simulink model "simThreeLinkFTC"  (R2014b)
settings: Solver=ode45  StartTime=0.0  StopTime=tof  FixedStep=dt  MaxStep=dtmax  RelTol=1e-3
values from neighbouring files (symbols this model uses):
  alpha = 1    [robotArmWith2Links.m]    (also in threeLinkFTC.m; twoLinkFTC.m; twoLinkFTCwAdaptive.m)
  Ar = [0 5; -30 -30]    [robotArmWith2Links.m]    (also in threeLinkFTC.m = [0 1; -5 -5]; twoLinkFTC.m = [0 10; -40 -40]; twoLinkFTCwAdaptive.m = [0 5; -250 -250])
  Arm1 = [0 1; -wn^2 -2*ksi*wn]    [robotArmWith2Links.m]    (also in threeLinkFTC.m; twoLinkFTC.m; twoLinkFTCwAdaptive.m)
  As = zeros(nofstates,nofstates)    [threeLinkFTC.m]    (also in twoLinkFDIbasisComparison.m; twoLinkFTC.m; twoLinkFTCwAdaptive.m)
  Brm1 = [0 wn^2]'    [robotArmWith2Links.m]    (also in threeLinkFTC.m; twoLinkFTC.m; twoLinkFTCwAdaptive.m)
  Dhat0 = zeros(6,1)    [threeLinkFTC.m]    (also in twoLinkFDIbasisComparison.m = zeros(4,1); twoLinkFTC.m = zeros(4,1); twoLinkFTCwAdaptive.m = zeros(4,1))
  Dlimit = 10    [threeLinkFTC.m]    (also in twoLinkFTC.m; twoLinkFTCwAdaptive.m)
  dtFc = 1*dtmax    (= 0.001)    [threeLinkFTC.m]    (also in twoLinkFDIbasisComparison.m; twoLinkFTC.m; twoLinkFTCwAdaptive.m)
  epsilon = 0.5    [robotArmWith2Links.m]    (also in threeLinkFTC.m; twoLinkFTC.m; twoLinkFTCwAdaptive.m)
  epsilontheta = 0.01    [threeLinkFTC.m]    (also in twoLinkFDIbasisComparison.m; twoLinkFTC.m; twoLinkFTCwAdaptive.m)
  faultyArm = 3    [threeLinkFTC.m]    (also in twoLinkFDIbasisComparison.m = 2; twoLinkFTC.m = 2; twoLinkFTCwAdaptive.m = 1)
  FDstart = 0.5    [threeLinkFTC.m]    (also in twoLinkFTC.m; twoLinkFTCwAdaptive.m)
  fmPosition = [0 90 -45]'*pi/180    [threeLinkFTC.m]    (also in twoLinkFTC.m = [90 0]'*pi/180; twoLinkFTCwAdaptive.m = [90 0]'*pi/180)
  g = 9.81    [robotArmWith2Links.m]    (also in threeLinkFTC.m; twoLinkFDIbasisComparison.m; twoLinkFTC.m; twoLinkFTCwAdaptive.m)
  GammaW = 1000    [threeLinkFTC.m]    (also in twoLinkFDIbasisComparison.m; twoLinkFTC.m; twoLinkFTCwAdaptive.m)
  I1 = 8.33e-2    (= 0.0833)    [robotArmWith2Links.m]    (also in threeLinkFTC.m = 0.0833333333333; twoLinkFDIbasisComparison.m = 0.0833333333333; twoLinkFTC.m = 0.0833333333333; twoLinkFTCwAdaptive.m = 0.0833333333333)
  I2 = 8.33e-2    (= 0.0833)    [robotArmWith2Links.m]    (also in threeLinkFTC.m = 0.0833333333333; twoLinkFDIbasisComparison.m = 0.0833333333333; twoLinkFTC.m = 0.0833333333333; twoLinkFTCwAdaptive.m = 0.0833333333333)
  I3 = m3*l3^2*1/12    (= 0.0833333333333)    [threeLinkFTC.m]
  ifault = 2    [threeLinkFTC.m]    (also in twoLinkFDIbasisComparison.m; twoLinkFTC.m; twoLinkFTCwAdaptive.m)
  K1 = 2*wn*ksi    (= 87.9645943005)    [robotArmWith2Links.m]    (also in threeLinkFTC.m = 8.79645943005; twoLinkFTC.m; twoLinkFTCwAdaptive.m = 43.9822971503)
  K2 = wn^2    (= 986.960440109)    [robotArmWith2Links.m]    (also in threeLinkFTC.m = 39.4784176044; twoLinkFTC.m; twoLinkFTCwAdaptive.m)
  Kp = wn^2    (= 157.913670417)    [threeLinkFTC.m]    (also in twoLinkFDIbasisComparison.m = 3947.84176044; twoLinkFTC.m = 3947.84176044; twoLinkFTCwAdaptive.m = 3947.84176044)
  Kv = 2*ksi*wn    (= 17.5929188601)    [threeLinkFTC.m]    (also in twoLinkFDIbasisComparison.m = 125.663706144; twoLinkFTC.m = 125.663706144; twoLinkFTCwAdaptive.m = 125.663706144)
  l1 = 1    [robotArmWith2Links.m]    (also in threeLinkFTC.m; twoLinkFDIbasisComparison.m; twoLinkFTC.m; twoLinkFTCwAdaptive.m)
  l2 = 1    [robotArmWith2Links.m]    (also in threeLinkFTC.m; twoLinkFDIbasisComparison.m; twoLinkFTC.m; twoLinkFTCwAdaptive.m)
  lc1 = l1/2    (= 0.5)    [robotArmWith2Links.m]    (also in threeLinkFTC.m; twoLinkFDIbasisComparison.m; twoLinkFTC.m; twoLinkFTCwAdaptive.m)
  lc2 = l2/2    (= 0.5)    [robotArmWith2Links.m]    (also in threeLinkFTC.m; twoLinkFDIbasisComparison.m; twoLinkFTC.m; twoLinkFTCwAdaptive.m)
  m1 = 1    [robotArmWith2Links.m]    (also in threeLinkFTC.m; twoLinkFDIbasisComparison.m; twoLinkFTC.m; twoLinkFTCwAdaptive.m)
  m2 = 1    [robotArmWith2Links.m]    (also in threeLinkFTC.m; twoLinkFDIbasisComparison.m; twoLinkFTC.m; twoLinkFTCwAdaptive.m)
  m3 = 1    [threeLinkFTC.m]
  nCheby = 4    [threeLinkFTC.m]    (also in twoLinkFDIbasisComparison.m; twoLinkFTC.m; twoLinkFTCwAdaptive.m)
  Ps = lyap(As(4:6,4:6)',Q)    [threeLinkFTC.m]    (also in twoLinkFDIbasisComparison.m = lyap(As(3:4,3:4)',Q); twoLinkFTC.m = lyap(As(3:4,3:4)',Q); twoLinkFTCwAdaptive.m = lyap(As(3:4,3:4)',Q))
  q0 = [80 20]'*pi/180    [robotArmWith2Links.m]    (also in threeLinkFTC.m = [90 0 0]'*pi/180; twoLinkFDIbasisComparison.m = [90 0]'*pi/180; twoLinkFTC.m = [90 0]'*pi/180; twoLinkFTCwAdaptive.m = [90 0]'*pi/180)
  qdot0 = [0 0]'    [robotArmWith2Links.m]    (also in threeLinkFTC.m = [0 0 0]'*pi/180; twoLinkFDIbasisComparison.m = [0 0]'*pi/180; twoLinkFTC.m = [0 0]'*pi/180; twoLinkFTCwAdaptive.m = [0 0]'*pi/180)
  r0 = [0 0]'    [robotArmWith2Links.m]    (also in threeLinkFTC.m; twoLinkFTC.m; twoLinkFTCwAdaptive.m)
  rmax = inf*[50*pi/180 inf]'    [robotArmWith2Links.m]    (also in threeLinkFTC.m; twoLinkFTC.m; twoLinkFTCwAdaptive.m)
  rmin = -rmax    [robotArmWith2Links.m]    (also in threeLinkFTC.m; twoLinkFTC.m; twoLinkFTCwAdaptive.m)
  tfault = 5    [threeLinkFTC.m]    (also in twoLinkFDIbasisComparison.m; twoLinkFTC.m; twoLinkFTCwAdaptive.m = 1)
  W0 = 0    [threeLinkFTC.m]    (also in twoLinkFDIbasisComparison.m; twoLinkFTC.m; twoLinkFTCwAdaptive.m)
  Wbnd = 1000    [threeLinkFTC.m]    (also in twoLinkFDIbasisComparison.m; twoLinkFTC.m; twoLinkFTCwAdaptive.m)
  xhat0 = [q0 ; qdot0]    [threeLinkFTC.m]    (also in twoLinkFDIbasisComparison.m; twoLinkFTC.m; twoLinkFTCwAdaptive.m)
undefined symbols (not defined in the file or in its folder): Intmax, Intmin
libraries: simulink x9, vrlib x3, dspbuff3 x1
(part 3 of 3)

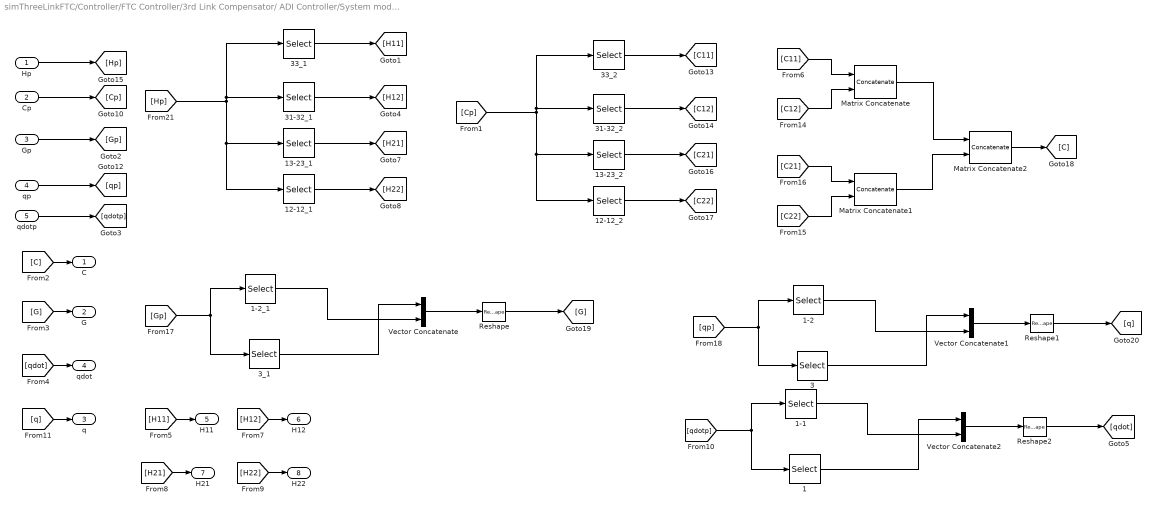
== system simThreeLinkFTC/Controller/FTC Controller/3rd Link Compensator/ ADI Controller/System model/Restructuring of System Matrices and States ==
  Hp : Inport
  Cp : Inport  Port=2
  Gp : Inport  Port=3
  qp : Inport  Port=4
  qdotp : Inport  Port=5
  1 : Selector  NumberOfDimensions=2  InputPortWidth=3  IndexOptions=Index vector (dialog),Index vector (dialog)  Indices=3,1  OutputSizes=1,1
  1-1 : Selector  NumberOfDimensions=2  InputPortWidth=3  IndexOptions=Index vector (dialog),Index vector (dialog)  Indices=[1 2],1  OutputSizes=1,1
  1-2 : Selector  NumberOfDimensions=2  InputPortWidth=3  IndexOptions=Index vector (dialog),Index vector (dialog)  Indices=[1 2],1  OutputSizes=1,1
  1-2_1 : Selector  NumberOfDimensions=2  InputPortWidth=3  IndexOptions=Index vector (dialog),Index vector (dialog)  Indices=[1 2],1  OutputSizes=1,1
  12-12_1 : Selector  NumberOfDimensions=2  InputPortWidth=3  IndexOptions=Index vector (dialog),Index vector (dialog)  Indices=[1 2],[1 2]  OutputSizes=1,1
  12-12_2 : Selector  NumberOfDimensions=2  InputPortWidth=3  IndexOptions=Index vector (dialog),Index vector (dialog)  Indices=[1 2],[1 2]  OutputSizes=1,1
  13-23_1 : Selector  NumberOfDimensions=2  InputPortWidth=3  IndexOptions=Index vector (dialog),Index vector (dialog)  Indices=[1 2],3  OutputSizes=1,1
  13-23_2 : Selector  NumberOfDimensions=2  InputPortWidth=3  IndexOptions=Index vector (dialog),Index vector (dialog)  Indices=[1 2],3  OutputSizes=1,1
  3 : Selector  NumberOfDimensions=2  InputPortWidth=3  IndexOptions=Index vector (dialog),Index vector (dialog)  Indices=3,1  OutputSizes=1,1
  31-32_1 : Selector  NumberOfDimensions=2  InputPortWidth=3  IndexOptions=Index vector (dialog),Index vector (dialog)  Indices=3,[1 2]  OutputSizes=1,1
  31-32_2 : Selector  NumberOfDimensions=2  InputPortWidth=3  IndexOptions=Index vector (dialog),Index vector (dialog)  Indices=3,[1 2]  OutputSizes=1,1
  33_1 : Selector  NumberOfDimensions=2  InputPortWidth=3  IndexOptions=Index vector (dialog),Index vector (dialog)  Indices=3,3  OutputSizes=1,1
  33_2 : Selector  NumberOfDimensions=2  InputPortWidth=3  IndexOptions=Index vector (dialog),Index vector (dialog)  Indices=3,3  OutputSizes=1,1
  3_1 : Selector  NumberOfDimensions=2  InputPortWidth=3  IndexOptions=Index vector (dialog),Index vector (dialog)  Indices=3,1  OutputSizes=1,1
  Matrix Concatenate : Concatenate  Mode=Multidimensional array  ConcatenateDimension=2
  Matrix Concatenate1 : Concatenate  Mode=Multidimensional array  ConcatenateDimension=2
  Matrix Concatenate2 : Concatenate  Mode=Multidimensional array
  Reshape : Reshape  OutputDimensionality=Column vector (2-D)
  Reshape1 : Reshape  OutputDimensionality=Column vector (2-D)
  Reshape2 : Reshape  OutputDimensionality=Column vector (2-D)
  Vector Concatenate : Concatenate
  Vector Concatenate1 : Concatenate
  Vector Concatenate2 : Concatenate
  C : Outport
  G : Outport  Port=2
  q : Outport  Port=3
  qdot : Outport  Port=4
  H11 : Outport  Port=5
  H12 : Outport  Port=6
  H21 : Outport  Port=7
  H22 : Outport  Port=8
  wires:
  [Hp] -> 33_1/1, 31-32_1/1, 13-23_1/1, 12-12_1/1
  12-12_1/1 -> [H22]
  31-32_1/1 -> [H12]
  33_1/1 -> [H11]
  13-23_1/1 -> [H21]
  12-12_2/1 -> [C22]
  Reshape1/1 -> [q]
  [Cp] -> 33_2/1, 31-32_2/1, 13-23_2/1, 12-12_2/1
  [C21] -> Matrix Concatenate1/1
  [C11] -> Matrix Concatenate/1
  Matrix Concatenate/1 -> Matrix Concatenate2/1
  [Gp] -> 3_1/1, 1-2_1/1
  Reshape/1 -> [G]
  Vector Concatenate/1 -> Reshape/1
  31-32_2/1 -> [C12]
  Matrix Concatenate1/1 -> Matrix Concatenate2/2
  1-2/1 -> Vector Concatenate1/2
  1-2_1/1 -> Vector Concatenate/2
  3/1 -> Vector Concatenate1/1
  13-23_2/1 -> [C21]
  [C12] -> Matrix Concatenate/2
  33_2/1 -> [C11]
  Matrix Concatenate2/1 -> [C]
  [C22] -> Matrix Concatenate1/2
  Vector Concatenate1/1 -> Reshape1/1
  3_1/1 -> Vector Concatenate/1
  [qp] -> 3/1, 1-2/1
  Cp/1 -> [Cp]
  Hp/1 -> [Hp]
  Gp/1 -> [Gp]
  qp/1 -> [qp]
  [C] -> C/1
  [G] -> G/1
  [qdot] -> qdot/1
  [H11] -> H11/1
  [H12] -> H12/1
  [H21] -> H21/1
  [H22] -> H22/1
  qdotp/1 -> [qdotp]
  Reshape2/1 -> [qdot]
  1-1/1 -> Vector Concatenate2/2
  1/1 -> Vector Concatenate2/1
  Vector Concatenate2/1 -> Reshape2/1
  [qdotp] -> 1-1/1, 1/1
  [q] -> q/1

== system simThreeLinkFTC/Controller/FTC Controller/3rd Link Compensator/Partial FBL q2 Controller/Torque calculation/Restructuring of System Matrices and States ==
  Hp : Inport
  Cp : Inport  Port=2
  Gp : Inport  Port=3
  qdotp : Inport  Port=4
  1-2 : Selector  NumberOfDimensions=2  InputPortWidth=3  IndexOptions=Index vector (dialog),Index vector (dialog)  Indices=[1 2],1  OutputSizes=1,1
  1-2_1 : Selector  NumberOfDimensions=2  InputPortWidth=3  IndexOptions=Index vector (dialog),Index vector (dialog)  Indices=[1 2],1  OutputSizes=1,1
  12-12_1 : Selector  NumberOfDimensions=2  InputPortWidth=3  IndexOptions=Index vector (dialog),Index vector (dialog)  Indices=[1 2],[1 2]  OutputSizes=1,1
  12-12_2 : Selector  NumberOfDimensions=2  InputPortWidth=3  IndexOptions=Index vector (dialog),Index vector (dialog)  Indices=[1 2],[1 2]  OutputSizes=1,1
  13-23_1 : Selector  NumberOfDimensions=2  InputPortWidth=3  IndexOptions=Index vector (dialog),Index vector (dialog)  Indices=[1 2],3  OutputSizes=1,1
  13-23_2 : Selector  NumberOfDimensions=2  InputPortWidth=3  IndexOptions=Index vector (dialog),Index vector (dialog)  Indices=[1 2],3  OutputSizes=1,1
  3 : Selector  NumberOfDimensions=2  InputPortWidth=3  IndexOptions=Index vector (dialog),Index vector (dialog)  Indices=3,1  OutputSizes=1,1
  31-32_1 : Selector  NumberOfDimensions=2  InputPortWidth=3  IndexOptions=Index vector (dialog),Index vector (dialog)  Indices=3,[1 2]  OutputSizes=1,1
  31-32_2 : Selector  NumberOfDimensions=2  InputPortWidth=3  IndexOptions=Index vector (dialog),Index vector (dialog)  Indices=3,[1 2]  OutputSizes=1,1
  33_1 : Selector  NumberOfDimensions=2  InputPortWidth=3  IndexOptions=Index vector (dialog),Index vector (dialog)  Indices=3,3  OutputSizes=1,1
  33_2 : Selector  NumberOfDimensions=2  InputPortWidth=3  IndexOptions=Index vector (dialog),Index vector (dialog)  Indices=3,3  OutputSizes=1,1
  3_1 : Selector  NumberOfDimensions=2  InputPortWidth=3  IndexOptions=Index vector (dialog),Index vector (dialog)  Indices=3,1  OutputSizes=1,1
  Matrix Concatenate : Concatenate  Mode=Multidimensional array  ConcatenateDimension=2
  Matrix Concatenate1 : Concatenate  Mode=Multidimensional array  ConcatenateDimension=2
  Matrix Concatenate2 : Concatenate  Mode=Multidimensional array
  Reshape : Reshape  OutputDimensionality=Column vector (2-D)
  Reshape1 : Reshape  OutputDimensionality=Column vector (2-D)
  Vector Concatenate : Concatenate
  Vector Concatenate1 : Concatenate
  C : Outport
  G : Outport  Port=2
  qdot : Outport  Port=3
  H11 : Outport  Port=4
  H12 : Outport  Port=5
  H21 : Outport  Port=6
  H22 : Outport  Port=7
  wires:
  [Hp] -> 33_1/1, 31-32_1/1, 13-23_1/1, 12-12_1/1
  12-12_1/1 -> [H22]
  31-32_1/1 -> [H12]
  33_1/1 -> [H11]
  13-23_1/1 -> [H21]
  12-12_2/1 -> [C22]
  Reshape1/1 -> [qdot]
  [Cp] -> 33_2/1, 31-32_2/1, 13-23_2/1, 12-12_2/1
  [C21] -> Matrix Concatenate1/1
  [C11] -> Matrix Concatenate/1
  Matrix Concatenate/1 -> Matrix Concatenate2/1
  [Gp] -> 3_1/1, 1-2_1/1
  Reshape/1 -> [G]
  Vector Concatenate/1 -> Reshape/1
  31-32_2/1 -> [C12]
  Matrix Concatenate1/1 -> Matrix Concatenate2/2
  1-2/1 -> Vector Concatenate1/2
  1-2_1/1 -> Vector Concatenate/2
  3/1 -> Vector Concatenate1/1
  13-23_2/1 -> [C21]
  [C12] -> Matrix Concatenate/2
  33_2/1 -> [C11]
  Matrix Concatenate2/1 -> [C]
  [C22] -> Matrix Concatenate1/2
  Vector Concatenate1/1 -> Reshape1/1
  3_1/1 -> Vector Concatenate/1
  [qdotp] -> 3/1, 1-2/1
  Cp/1 -> [Cp]
  Hp/1 -> [Hp]
  Gp/1 -> [Gp]
  qdotp/1 -> [qdotp]
  [C] -> C/1
  [G] -> G/1
  [qdot] -> qdot/1
  [H11] -> H11/1
  [H12] -> H12/1
  [H21] -> H21/1
  [H22] -> H22/1

== system simThreeLinkFTC/Controller/FTC Controller/1st Link Compensator/ ADI Controller/System model/Modelled Plant/get Plant Parameters ==
  H : Inport
  C : Inport  Port=2
  G : Inport  Port=3
  qdot : Inport  Port=4
  {1,5,7,11} (4 alike) : Selector  NumberOfDimensions=2  InputPortWidth=3  IndexOptions=Index vector (dialog),Index vector (dialog)  Indices=1,1  OutputSizes=1,1
  12 : Selector  NumberOfDimensions=2  InputPortWidth=3  IndexOptions=Index vector (dialog),Index vector (dialog)  Indices=1,2  OutputSizes=1,1
  2 : Selector  NumberOfDimensions=2  InputPortWidth=3  IndexOptions=Index vector (dialog),Index vector (dialog)  Indices=1,2  OutputSizes=1,1
  {3,6,8,21} (4 alike) : Selector  NumberOfDimensions=2  InputPortWidth=3  IndexOptions=Index vector (dialog),Index vector (dialog)  Indices=2,1  OutputSizes=1,1
  22 : Selector  NumberOfDimensions=2  InputPortWidth=3  IndexOptions=Index vector (dialog),Index vector (dialog)  Indices=2,2  OutputSizes=1,1
  4 : Selector  NumberOfDimensions=2  InputPortWidth=3  IndexOptions=Index vector (dialog),Index vector (dialog)  Indices=2,2  OutputSizes=1,1
  Bus Creator : BusCreator  Inputs=15
  Product5 : Product  Multiplication=Matrix(*)  RndMeth=Zero
  Sum of Elements1 : Sum
  busData : Outport
  wires:
  qdot/1 -> [qdot]
  G/1 -> [G]  "G"
  C/1 -> [C]  "C"
  H/1 -> [H]  "H"
  [H] -> Bus Creator/1
  [C] -> Bus Creator/2
  Bus Creator/1 -> busData/1
  [G] -> Bus Creator/3
  8/1 -> Bus Creator/15  "phi2"
  7/1 -> Bus Creator/14  "phi1"
  Sum of Elements1/1 -> 8/1, 7/1
  [G] -> Sum of Elements1/2
  Product5/1 -> Sum of Elements1/1
  [qdot] -> Product5/2
  [C] -> Product5/1
  [G] -> 5/1, 6/1
  [C] -> 3/1, 4/1, 2/1, 1/1
  [H] -> 22/1, 21/1, 12/1, 11/1
  11/1 -> Bus Creator/4  "H11"
  3/1 -> Bus Creator/10  "C21"
  12/1 -> Bus Creator/5  "H12"
  5/1 -> Bus Creator/12  "G_1"
  1/1 -> Bus Creator/8  "C11"
  6/1 -> Bus Creator/13  "G_2"
  4/1 -> Bus Creator/11  "C22"
  22/1 -> Bus Creator/7  "H22"
  21/1 -> Bus Creator/6  "H21"
  2/1 -> Bus Creator/9  "C12"

== system simThreeLinkFTC/Controller/FTC Controller/1st Link Compensator/ ADI Controller/System model/Modelled Plant/getC ==
  s2 : Inport
  q1dot : Inport  Port=2
  q2dot : Inport  Port=3
  C calculation 1 : Subsystem
  C calculation 2 : Subsystem
  Gain2 : Gain  Gain=m2*l1*lc2
  Terminator : Terminator
  C : Outport
  wires:
  C calculation 1/1(C) -> Terminator/1
  C calculation 2/1(C) -> [C]
  [C] -> C/1
  [h] -> C calculation 2/3(h)
  [q2dot] -> C calculation 2/2(q2dot)
  [q1dot] -> C calculation 2/1(q1dot)
  [h] -> C calculation 1/3(h)
  [q2dot] -> C calculation 1/2(q2dot)
  [q1dot] -> C calculation 1/1(q1dot)
  Gain2/1 -> [h]
  [s2] -> Gain2/1
  q2dot/1 -> [q2dot]
  q1dot/1 -> [q1dot]
  s2/1 -> [s2]

== system simThreeLinkFTC/Controller/FTC Controller/1st Link Compensator/ ADI Controller/System model/Modelled Plant/getG ==
  c1 : Inport
  c12 : Inport  Port=2
  Add : Sum
  Gain : Gain  Gain=(m1*lc1+m2*l1)*g
  Gain1 : Gain  Gain=m2*g*lc2
  Gain2 : Gain
  Gain4 : Gain  Gain=lc2*m2*g
  Matrix Concatenate2 : Concatenate  Mode=Multidimensional array
  G : Outport
  wires:
  Gain2/1 -> G/1
  Add/1 -> [G11]
  Gain1/1 -> Add/2
  [c12] -> Gain1/1
  Gain/1 -> Add/1
  [c1] -> Gain/1
  [G21] -> Matrix Concatenate2/2
  [G11] -> Matrix Concatenate2/1
  Matrix Concatenate2/1 -> Gain2/1
  c1/1 -> [c1]
  c12/1 -> [c12]
  Gain4/1 -> [G21]
  [c12] -> Gain4/1

== system simThreeLinkFTC/Controller/FTC Controller/1st Link Compensator/ ADI Controller/System model/Modelled Plant/getH ==
  c2 : Inport
  Constant1 : Constant  Value=I1 + I2 + m1*lc1^2 + m2*(l1^2+lc2^2)  VectorParams1D=off
  Constant2 : Constant  Value=I2+m2*lc2^2  VectorParams1D=off
  Constant3 : Constant  Value=I2+m2*lc2^2  VectorParams1D=off
  Gain : Gain  Gain=m2*2*l1*lc2
  Gain1 : Gain  Gain=m2*l1*lc2
  Matrix Concatenate : Concatenate  Mode=Multidimensional array  ConcatenateDimension=2
  Matrix Concatenate1 : Concatenate  Mode=Multidimensional array  ConcatenateDimension=2
  Matrix Concatenate2 : Concatenate  Mode=Multidimensional array
  Sum : Sum
  Sum1 : Sum
  H : Outport
  wires:
  Constant3/1 -> [H22]
  Sum1/1 -> [H21], [H12]
  Constant2/1 -> Sum1/2
  Gain1/1 -> Sum1/1
  [c2] -> Gain1/1
  Sum/1 -> [H11]
  Constant1/1 -> Sum/2
  Gain/1 -> Sum/1
  [c2] -> Gain/1
  c2/1 -> [c2]
  Matrix Concatenate2/1 -> H/1
  [H22] -> Matrix Concatenate1/2
  [H21] -> Matrix Concatenate1/1
  Matrix Concatenate1/1 -> Matrix Concatenate2/2
  Matrix Concatenate/1 -> Matrix Concatenate2/1
  [H12] -> Matrix Concatenate/2
  [H11] -> Matrix Concatenate/1

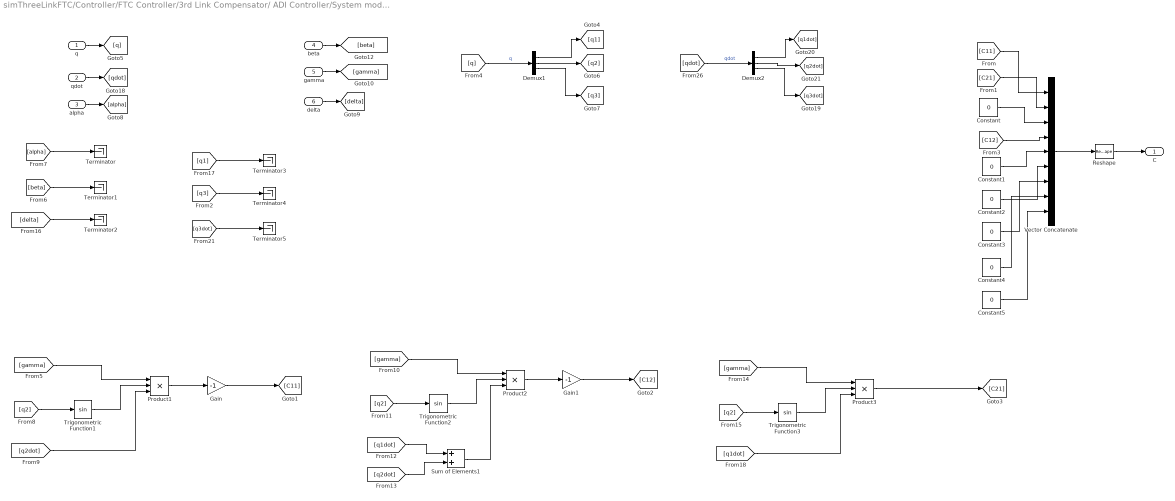
== system simThreeLinkFTC/Controller/FTC Controller/3rd Link Compensator/ ADI Controller/System model/Modelled Plant/getC ==
  q : Inport
  qdot : Inport  Port=2
  alpha : Inport  Port=3
  beta : Inport  Port=4
  gamma : Inport  Port=5
  delta : Inport  Port=6
  Constant{,1..5} (6 alike) : Constant  Value=0  VectorParams1D=off
  Demux1 : Demux  Outputs=3
  Demux2 : Demux  Outputs=3
  Gain : Gain  Gain=-1
  Gain1 : Gain  Gain=-1
  Product1 : Product  Inputs=3
  Product2 : Product  Inputs=3
  Product3 : Product  Inputs=3
  Reshape : Reshape  OutputDimensionality=Customize  OutputDimensions=[3,3]
  Sum of Elements1 : Sum
  Terminator{,1..5} (6 alike) : Terminator
  Trigonometric Function1 : Trigonometry
  Trigonometric Function2 : Trigonometry
  Trigonometric Function3 : Trigonometry
  Vector Concatenate : Concatenate  NumInputs=9
  C : Outport
  wires:
  [C11] -> Vector Concatenate/1
  [C21] -> Vector Concatenate/2
  Constant/1 -> Vector Concatenate/3
  Constant1/1 -> Vector Concatenate/5
  [C12] -> Vector Concatenate/4
  Vector Concatenate/1 -> Reshape/1
  beta/1 -> [beta]
  gamma/1 -> [gamma]
  delta/1 -> [delta]
  alpha/1 -> [alpha]
  Demux1/2 -> [q2]
  Demux1/3 -> [q3]
  Demux1/1 -> [q1]
  [q] -> Demux1/1  "q"
  q/1 -> [q]
  Reshape/1 -> C/1
  qdot/1 -> [qdot]
  [qdot] -> Demux2/1  "qdot"
  Demux2/1 -> [q1dot]
  Demux2/3 -> [q3dot]
  Demux2/2 -> [q2dot]
  Constant2/1 -> Vector Concatenate/6
  Constant3/1 -> Vector Concatenate/7
  Constant4/1 -> Vector Concatenate/8
  Constant5/1 -> Vector Concatenate/9
  [q3dot] -> Terminator5/1
  [q3] -> Terminator4/1
  [q1] -> Terminator3/1
  [alpha] -> Terminator/1
  [beta] -> Terminator1/1
  [delta] -> Terminator2/1
  [q2] -> Trigonometric Function1/1
  [gamma] -> Product1/1
  Trigonometric Function1/1 -> Product1/2
  [q2dot] -> Product1/3
  Product1/1 -> Gain/1
  Gain/1 -> [C11]
  [q2] -> Trigonometric Function2/1
  [gamma] -> Product2/1
  Trigonometric Function2/1 -> Product2/2
  Product2/1 -> Gain1/1
  Gain1/1 -> [C12]
  [q1dot] -> Sum of Elements1/1
  [q2dot] -> Sum of Elements1/2
  Sum of Elements1/1 -> Product2/3
  [q2] -> Trigonometric Function3/1
  [gamma] -> Product3/1
  Trigonometric Function3/1 -> Product3/2
  [q1dot] -> Product3/3
  Product3/1 -> [C21]

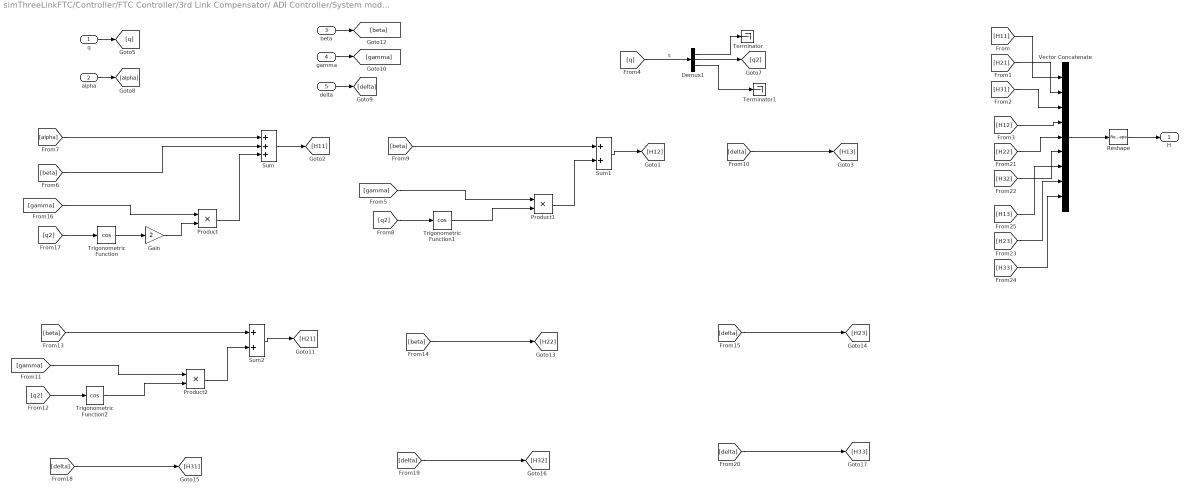
== system simThreeLinkFTC/Controller/FTC Controller/3rd Link Compensator/ ADI Controller/System model/Modelled Plant/getH ==
  q : Inport
  alpha : Inport  Port=2
  beta : Inport  Port=3
  gamma : Inport  Port=4
  delta : Inport  Port=5
  Demux1 : Demux  Outputs=3
  Gain : Gain  Gain=2
  Product : Product
  Product1 : Product
  Product2 : Product
  Reshape : Reshape  OutputDimensionality=Customize  OutputDimensions=[3,3]
  Sum : Sum  Inputs=+++
  Sum1 : Sum
  Sum2 : Sum
  Terminator : Terminator
  Terminator1 : Terminator
  Trigonometric Function : Trigonometry  Operator=cos
  Trigonometric Function1 : Trigonometry  Operator=cos
  Trigonometric Function2 : Trigonometry  Operator=cos
  Vector Concatenate : Concatenate  NumInputs=9
  H : Outport
  wires:
  Reshape/1 -> H/1
  Sum/1 -> [H11]
  q/1 -> [q]
  [q] -> Demux1/1  "q"
  Demux1/1 -> Terminator/1
  Demux1/2 -> [q2]
  alpha/1 -> [alpha]
  delta/1 -> [delta]
  gamma/1 -> [gamma]
  beta/1 -> [beta]
  [q2] -> Trigonometric Function/1
  Trigonometric Function/1 -> Gain/1
  [gamma] -> Product/1
  Gain/1 -> Product/2
  [alpha] -> Sum/1
  [beta] -> Sum/2
  Product/1 -> Sum/3
  Sum1/1 -> [H12]
  [q2] -> Trigonometric Function1/1
  [gamma] -> Product1/1
  Trigonometric Function1/1 -> Product1/2
  [beta] -> Sum1/1
  Product1/1 -> Sum1/2
  [delta] -> [H13]
  Sum2/1 -> [H21]
  [q2] -> Trigonometric Function2/1
  [gamma] -> Product2/1
  Trigonometric Function2/1 -> Product2/2
  [beta] -> Sum2/1
  Product2/1 -> Sum2/2
  [beta] -> [H22]
  [delta] -> [H23]
  [delta] -> [H31]
  [delta] -> [H32]
  [delta] -> [H33]
  Vector Concatenate/1 -> Reshape/1
  [H12] -> Vector Concatenate/4
  [H22] -> Vector Concatenate/5
  [H31] -> Vector Concatenate/3
  [H32] -> Vector Concatenate/6
  [H21] -> Vector Concatenate/2
  [H11] -> Vector Concatenate/1
  [H13] -> Vector Concatenate/7
  [H23] -> Vector Concatenate/8
  [H33] -> Vector Concatenate/9
  Demux1/3 -> Terminator1/1

== system simThreeLinkFTC/Controller/FTC Controller/1st Link Compensator/ ADI Controller/System model/Modelled Plant/getC/C calculation 1 ==
  q1dot : Inport
  q2dot : Inport  Port=2
  h : Inport  Port=3
  Constant3 : Constant  Value=0  VectorParams1D=off
  Gain2 : Gain  Gain=-1
  Gain3 : Gain  Gain=-1
  Gain5 : Gain  Gain=-1
  Matrix Concatenate : Concatenate  Mode=Multidimensional array  ConcatenateDimension=2
  Matrix Concatenate1 : Concatenate  Mode=Multidimensional array  ConcatenateDimension=2
  Matrix Concatenate2 : Concatenate  Mode=Multidimensional array
  Product{,1..7} (8 alike) : Product  RndMeth=Zero
  Sum{,1..3} (4 alike) : Sum
  C : Outport
  wires:
  [C11] -> Matrix Concatenate/1
  [C12] -> Matrix Concatenate/2
  Matrix Concatenate/1 -> Matrix Concatenate2/1
  Matrix Concatenate1/1 -> Matrix Concatenate2/2
  [C21] -> Matrix Concatenate1/1
  [C22] -> Matrix Concatenate1/2
  Matrix Concatenate2/1 -> C/1
  Sum3/1 -> [C22]
  h/1 -> [h]
  Gain5/1 -> [N122]
  Gain3/1 -> [N121]
  Gain2/1 -> [N112]
  [h] -> [N211], Gain5/1, Gain3/1, Gain2/1
  Constant3/1 -> [N222], [N221], [N212], [N111]
  [q2dot] -> Product7/2
  Product7/1 -> Sum3/2
  [N222] -> Product7/1
  [q1dot] -> Product5/2
  Product5/1 -> Sum3/1
  [N221] -> Product5/1
  Sum2/1 -> [C21]
  [q2dot] -> Product6/2
  Product6/1 -> Sum2/2
  [N212] -> Product6/1
  [q1dot] -> Product4/2
  Product4/1 -> Sum2/1
  [N211] -> Product4/1
  Sum1/1 -> [C12]
  [q2dot] -> Product3/2
  Product3/1 -> Sum1/2
  [N122] -> Product3/1
  [q1dot] -> Product1/2
  Product1/1 -> Sum1/1
  [N121] -> Product1/1
  Sum/1 -> [C11]
  [q2dot] -> Product2/2
  Product2/1 -> Sum/2
  [N112] -> Product2/1
  [q1dot] -> Product/2
  Product/1 -> Sum/1
  [N111] -> Product/1
  q1dot/1 -> [q1dot]
  q2dot/1 -> [q2dot]

== system simThreeLinkFTC/Controller/FTC Controller/1st Link Compensator/ ADI Controller/System model/Modelled Plant/getC/C calculation 2 ==
  q1dot : Inport
  q2dot : Inport  Port=2
  h : Inport  Port=3
  Constant1 : Constant  Value=0  VectorParams1D=off
  Gain6 : Gain  Gain=-2
  Gain7 : Gain  Gain=-1
  Matrix Concatenate : Concatenate  Mode=Multidimensional array  ConcatenateDimension=2
  Matrix Concatenate1 : Concatenate  Mode=Multidimensional array  ConcatenateDimension=2
  Matrix Concatenate2 : Concatenate  Mode=Multidimensional array
  Product10 : Product  RndMeth=Zero
  Product8 : Product  RndMeth=Zero
  Product9 : Product  RndMeth=Zero
  C : Outport
  wires:
  [q2dot] -> Product10/1
  [C11] -> Matrix Concatenate/1
  [C12] -> Matrix Concatenate/2
  Matrix Concatenate/1 -> Matrix Concatenate2/1
  Matrix Concatenate1/1 -> Matrix Concatenate2/2
  [C21] -> Matrix Concatenate1/1
  [C22] -> Matrix Concatenate1/2
  Matrix Concatenate2/1 -> C/1
  [q2dot] -> Product9/1
  Product9/1 -> [C11]
  Gain6/1 -> Product9/2
  Product8/1 -> [C21]
  [q1dot] -> Product8/1
  [h] -> Product8/2
  Constant1/1 -> [C22]
  Product10/1 -> [C12]
  Gain7/1 -> Product10/2
  [h] -> Gain7/1
  [h] -> Gain6/1
  q2dot/1 -> [q2dot]
  q1dot/1 -> [q1dot]
  h/1 -> [h]
